simulink model "Computed_Torque_Control"  (R2018b)
settings: Solver=FixedStepAuto  StartTime=0.0  StopTime=5  FixedStep=0.0005  RelTol=1e-3
model workspace (MAT data in the model file):
  Ball.radius = 0.03
  Ball.density = 1000
  Plane.length = 1
  Plane.width = 1
  Plane.depth = 0.1
  SCARA_Robot = robotics.RigidBodyTree
  SCARA_Robot.TreeInternal = robotics.manip.internal.RigidBodyTree
  SCARA_Robot.TreeInternal.NumBodies = 7
  SCARA_Robot.TreeInternal.Base = robotics.manip.internal.RigidBody
  SCARA_Robot.TreeInternal.Base.Index = 0
  SCARA_Robot.TreeInternal.Base.NameInternal = 'Base'
  SCARA_Robot.TreeInternal.Base.JointInternal = robotics.Joint
  SCARA_Robot.TreeInternal.Base.JointInternal.Type = 'fixed'
  SCARA_Robot.TreeInternal.Base.JointInternal.VelocityNumber = 0
  SCARA_Robot.TreeInternal.Base.JointInternal.PositionNumber = 0
  SCARA_Robot.TreeInternal.Base.JointInternal.MotionSubspace = [0; 0; 0; 0; 0; 0]
  SCARA_Robot.TreeInternal.Base.JointInternal.NameInternal = 'base_jnt'
  SCARA_Robot.TreeInternal.Base.ParentIndex = -1
  SCARA_Robot.TreeInternal.Base.ChildrenIndices = [1 0 0 0 0 0 1]
  SCARA_Robot.TreeInternal.Base.MassInternal = 1
  SCARA_Robot.TreeInternal.Base.CenterOfMassInternal = [0 0 0]
  SCARA_Robot.TreeInternal.Base.InertiaInternal = [1  0  0; 0  1  0; 0  0  1]
  SCARA_Robot.TreeInternal.Base.SpatialInertia = [1  0  0  0  0  0; 0  1  0  0  0  0; 0  0  1  0  0  0; 0  0  0  1  0  0; 0  0  0  0  1  0; 0  0  0  0  0  1]
  SCARA_Robot.TreeInternal.Gravity = [0 0 -9.80665]
  SCARA_Robot.TreeInternal.Bodies{1} = robotics.manip.internal.RigidBody
  SCARA_Robot.TreeInternal.Bodies{1}.Index = 1
  SCARA_Robot.TreeInternal.Bodies{1}.NameInternal = 'Body1'
  SCARA_Robot.TreeInternal.Bodies{1}.JointInternal = robotics.Joint
  SCARA_Robot.TreeInternal.Bodies{1}.JointInternal.Type = 'revolute'
  SCARA_Robot.TreeInternal.Bodies{1}.JointInternal.VelocityNumber = 1
  SCARA_Robot.TreeInternal.Bodies{1}.JointInternal.PositionNumber = 1
  SCARA_Robot.TreeInternal.Bodies{1}.JointInternal.MotionSubspace = [0; 0; 1; 0; 0; 0]
  SCARA_Robot.TreeInternal.Bodies{1}.JointInternal.InTree = 1
  SCARA_Robot.TreeInternal.Bodies{1}.JointInternal.JointToParentTransform = [1  0  0  0; 0  1  0  0; 0  0  1  0.2335; 0  0  0  1]
  SCARA_Robot.TreeInternal.Bodies{1}.JointInternal.NameInternal = 'Joint1'
  SCARA_Robot.TreeInternal.Bodies{1}.JointInternal.PositionLimitsInternal = [-3.14159265359 3.14159265359]
  SCARA_Robot.TreeInternal.Bodies{1}.JointInternal.JointAxisInternal = [0 0 1]
  SCARA_Robot.TreeInternal.Bodies{1}.ParentIndex = 0
  SCARA_Robot.TreeInternal.Bodies{1}.ChildrenIndices = [0 1]
  SCARA_Robot.TreeInternal.Bodies{1}.MassInternal = 3.12934702863
  SCARA_Robot.TreeInternal.Bodies{1}.CenterOfMassInternal = [0.108937389495 0 0.0763962080079]
  SCARA_Robot.TreeInternal.Bodies{1}.InertiaInternal = [0.0248122549552  -1.93363586828e-20  -0.0276846659585; -1.93363586828e-20  0.092692509819  4.00877355014e-19; -0.0276846659585  4.00877355014e-19  0.0776265146367]
  SCARA_Robot.TreeInternal.Bodies{1}.SpatialInertia = [0.0248122549552  -1.93363586828e-20  -0.0276846659585  0  -0.239070246528  0; -1.93363586828e-20  0.092692509819  4.00877355014e-19  0.239070246528  0  -0.340902896122; -0.0276846659585  4.00877355014e-19  0.0776265146367  0  0.340902896122  0; 0  0.239070246528  0  3.12934702863  0  0; -0.239070246528  0  0.340902896122  0  3.12934702863  0; 0  -0.340902896122  0  0  0  3.12934702863]
  SCARA_Robot.TreeInternal.Bodies{2} = robotics.manip.internal.RigidBody
  SCARA_Robot.TreeInternal.Bodies{2}.Index = 2
  SCARA_Robot.TreeInternal.Bodies{2}.NameInternal = 'Body2'
  SCARA_Robot.TreeInternal.Bodies{2}.JointInternal = robotics.Joint
  SCARA_Robot.TreeInternal.Bodies{2}.JointInternal.Type = 'revolute'
  SCARA_Robot.TreeInternal.Bodies{2}.JointInternal.VelocityNumber = 1
  SCARA_Robot.TreeInternal.Bodies{2}.JointInternal.PositionNumber = 1
  SCARA_Robot.TreeInternal.Bodies{2}.JointInternal.MotionSubspace = [0; 0; 1; 0; 0; 0]
  SCARA_Robot.TreeInternal.Bodies{2}.JointInternal.InTree = 1
  SCARA_Robot.TreeInternal.Bodies{2}.JointInternal.JointToParentTransform = [1  0  0  0.25; 0  1  0  0; 0  0  1  0.09; 0  0  0  1]
  SCARA_Robot.TreeInternal.Bodies{2}.JointInternal.NameInternal = 'Joint2'
  SCARA_Robot.TreeInternal.Bodies{2}.JointInternal.PositionLimitsInternal = [-3.14159265359 3.14159265359]
  SCARA_Robot.TreeInternal.Bodies{2}.JointInternal.JointAxisInternal = [0 0 1]
  SCARA_Robot.TreeInternal.Bodies{2}.ParentIndex = 1
  SCARA_Robot.TreeInternal.Bodies{2}.ChildrenIndices = [0 0 1]
  SCARA_Robot.TreeInternal.Bodies{2}.MassInternal = 2.8
  SCARA_Robot.TreeInternal.Bodies{2}.CenterOfMassInternal = [0.0730251626831 0 0.08]
  SCARA_Robot.TreeInternal.Bodies{2}.InertiaInternal = [0.0343024465413  9.77217250727e-20  -0.016902140627; 9.77217250727e-20  0.0618863054598  -9.17919345749e-19; -0.016902140627  -9.17919345749e-19  0.0363706015866]
  SCARA_Robot.TreeInternal.Bodies{2}.SpatialInertia = [0.0343024465413  9.77217250727e-20  -0.016902140627  0  -0.224  0; 9.77217250727e-20  0.0618863054598  -9.17919345749e-19  0.224  0  -0.204470455513; -0.016902140627  -9.17919345749e-19  0.0363706015866  0  0.204470455513  0; 0  0.224  0  2.8  0  0; -0.224  0  0.204470455513  0  2.8  0; 0  -0.204470455513  0  0  0  2.8]
  SCARA_Robot.TreeInternal.Bodies{3} = robotics.manip.internal.RigidBody
  SCARA_Robot.TreeInternal.Bodies{3}.Index = 3
  SCARA_Robot.TreeInternal.Bodies{3}.NameInternal = 'Body3'
  SCARA_Robot.TreeInternal.Bodies{3}.JointInternal = robotics.Joint
  SCARA_Robot.TreeInternal.Bodies{3}.JointInternal.Type = 'prismatic'
  SCARA_Robot.TreeInternal.Bodies{3}.JointInternal.VelocityNumber = 1
  SCARA_Robot.TreeInternal.Bodies{3}.JointInternal.PositionNumber = 1
  SCARA_Robot.TreeInternal.Bodies{3}.JointInternal.MotionSubspace = [0; 0; 0; 0; 0; 1]
  SCARA_Robot.TreeInternal.Bodies{3}.JointInternal.InTree = 1
  SCARA_Robot.TreeInternal.Bodies{3}.JointInternal.JointToParentTransform = [1  0  0  0.142; 0  1  0  -0.008; 0  0  1  0.25; 0  0  0  1]
  SCARA_Robot.TreeInternal.Bodies{3}.JointInternal.NameInternal = 'Joint3'
  SCARA_Robot.TreeInternal.Bodies{3}.JointInternal.PositionLimitsInternal = [-0.5 0.5]
  SCARA_Robot.TreeInternal.Bodies{3}.JointInternal.JointAxisInternal = [0 0 1]
  SCARA_Robot.TreeInternal.Bodies{3}.ParentIndex = 2
  SCARA_Robot.TreeInternal.Bodies{3}.ChildrenIndices = [0 0 0 1]
  SCARA_Robot.TreeInternal.Bodies{3}.MassInternal = 0.0658123859659
  SCARA_Robot.TreeInternal.Bodies{3}.CenterOfMassInternal = [0.008 0.008 -0.161652320553]
  SCARA_Robot.TreeInternal.Bodies{3}.InertiaInternal = [0.00223249562485  -4.21199270182e-06  8.51097993001e-05; -4.21199270182e-06  0.00223249562485  8.51097993001e-05; 8.51097993001e-05  8.51097993001e-05  1.08030484212e-05]
  SCARA_Robot.TreeInternal.Bodies{3}.SpatialInertia = [0.00223249562485  -4.21199270182e-06  8.51097993001e-05  0  0.0106387249125  0.000526499087728; -4.21199270182e-06  0.00223249562485  8.51097993001e-05  -0.0106387249125  0  -0.000526499087728; 8.51097993001e-05  8.51097993001e-05  1.08030484212e-05  -0.000526499087728  0.000526499087728  0; 0  -0.0106387249125  -0.000526499087728  0.0658123859659  0  0; 0.0106387249125  0  0.000526499087728  0  0.0658123859659  0; 0.000526499087728  -0.000526499087728  0  0  0  0.0658123859659]
  SCARA_Robot.TreeInternal.Bodies{4} = robotics.manip.internal.RigidBody
  SCARA_Robot.TreeInternal.Bodies{4}.Index = 4
  SCARA_Robot.TreeInternal.Bodies{4}.NameInternal = 'Body4'
  SCARA_Robot.TreeInternal.Bodies{4}.JointInternal = robotics.Joint
  SCARA_Robot.TreeInternal.Bodies{4}.JointInternal.Type = 'revolute'
  SCARA_Robot.TreeInternal.Bodies{4}.JointInternal.VelocityNumber = 1
  SCARA_Robot.TreeInternal.Bodies{4}.JointInternal.PositionNumber = 1
  SCARA_Robot.TreeInternal.Bodies{4}.JointInternal.MotionSubspace = [0; 0; 1; 0; 0; 0]
  SCARA_Robot.TreeInternal.Bodies{4}.JointInternal.InTree = 1
  SCARA_Robot.TreeInternal.Bodies{4}.JointInternal.JointToParentTransform = [1  0  0  0.008; 0  1  0  0.008; 0  0  1  -0.02; 0  0  0  1]
  SCARA_Robot.TreeInternal.Bodies{4}.JointInternal.NameInternal = 'Joint4'
  SCARA_Robot.TreeInternal.Bodies{4}.JointInternal.PositionLimitsInternal = [-3.14159265359 3.14159265359]
  SCARA_Robot.TreeInternal.Bodies{4}.JointInternal.JointAxisInternal = [0 0 1]
  SCARA_Robot.TreeInternal.Bodies{4}.ParentIndex = 3
  SCARA_Robot.TreeInternal.Bodies{4}.ChildrenIndices = [0 0 0 0 1]
  SCARA_Robot.TreeInternal.Bodies{4}.MassInternal = 0.0638828919245
  SCARA_Robot.TreeInternal.Bodies{4}.CenterOfMassInternal = [-0.000115977158264 0 -0.314685264828]
  SCARA_Robot.TreeInternal.Bodies{4}.InertiaInternal = [0.00634242429346  0  -2.33382122413e-06; 0  0.0063422366579  0; -2.33382122413e-06  0  2.29864595889e-05]
  SCARA_Robot.TreeInternal.Bodies{4}.SpatialInertia = [0.00634242429346  0  -2.33382122413e-06  0  0.0201030047632  0; 0  0.0063422366579  0  -0.0201030047632  0  7.40895626708e-06; -2.33382122413e-06  0  2.29864595889e-05  0  -7.40895626708e-06  0; 0  -0.0201030047632  0  0.0638828919245  0  0; 0.0201030047632  0  -7.40895626708e-06  0  0.0638828919245  0; 0  7.40895626708e-06  0  0  0  0.0638828919245]
  SCARA_Robot.TreeInternal.Bodies{5} = robotics.manip.internal.RigidBody
  SCARA_Robot.TreeInternal.Bodies{5}.Index = 5
  SCARA_Robot.TreeInternal.Bodies{5}.NameInternal = 'Body5'
  SCARA_Robot.TreeInternal.Bodies{5}.JointInternal = robotics.Joint
  SCARA_Robot.TreeInternal.Bodies{5}.JointInternal.Type = 'fixed'
  SCARA_Robot.TreeInternal.Bodies{5}.JointInternal.VelocityNumber = 0
  SCARA_Robot.TreeInternal.Bodies{5}.JointInternal.PositionNumber = 0
  SCARA_Robot.TreeInternal.Bodies{5}.JointInternal.MotionSubspace = [0; 0; 0; 0; 0; 0]
  SCARA_Robot.TreeInternal.Bodies{5}.JointInternal.InTree = 1
  SCARA_Robot.TreeInternal.Bodies{5}.JointInternal.JointToParentTransform = [1  0  0  -2.71050543121e-20; 0  1  0  0; 0  0  1  -0.33; 0  0  0  1]
  SCARA_Robot.TreeInternal.Bodies{5}.JointInternal.NameInternal = 'Joint5'
  SCARA_Robot.TreeInternal.Bodies{5}.ParentIndex = 4
  SCARA_Robot.TreeInternal.Bodies{5}.ChildrenIndices = [0 0 0 0 0 1]
  SCARA_Robot.TreeInternal.Bodies{5}.MassInternal = 0
  SCARA_Robot.TreeInternal.Bodies{5}.CenterOfMassInternal = [0 0 0]
  SCARA_Robot.TreeInternal.Bodies{5}.InertiaInternal = [0  0  0; 0  0  0; 0  0  0]
  SCARA_Robot.TreeInternal.Bodies{5}.SpatialInertia = [0  0  0  0  0  0; 0  0  0  0  0  0; 0  0  0  0  0  0; 0  0  0  0  0  0; 0  0  0  0  0  0; 0  0  0  0  0  0]
  SCARA_Robot.TreeInternal.Bodies{6} = robotics.manip.internal.RigidBody
  SCARA_Robot.TreeInternal.Bodies{6}.Index = 6
  SCARA_Robot.TreeInternal.Bodies{6}.NameInternal = 'Body6'
  SCARA_Robot.TreeInternal.Bodies{6}.JointInternal = robotics.Joint
  SCARA_Robot.TreeInternal.Bodies{6}.JointInternal.Type = 'fixed'
  SCARA_Robot.TreeInternal.Bodies{6}.JointInternal.VelocityNumber = 0
  SCARA_Robot.TreeInternal.Bodies{6}.JointInternal.PositionNumber = 0
  SCARA_Robot.TreeInternal.Bodies{6}.JointInternal.MotionSubspace = [0; 0; 0; 0; 0; 0]
  SCARA_Robot.TreeInternal.Bodies{6}.JointInternal.InTree = 1
  SCARA_Robot.TreeInternal.Bodies{6}.JointInternal.JointToParentTransform = [1  0  0  0; 0  1  0  0; 0  0  1  0; 0  0  0  1]
  SCARA_Robot.TreeInternal.Bodies{6}.JointInternal.NameInternal = 'Joint6'
  SCARA_Robot.TreeInternal.Bodies{6}.ParentIndex = 5
  SCARA_Robot.TreeInternal.Bodies{6}.ChildrenIndices = [0 0 0 0 0]
  SCARA_Robot.TreeInternal.Bodies{6}.MassInternal = 0.113097335529
  SCARA_Robot.TreeInternal.Bodies{6}.CenterOfMassInternal = [0 0 0]
  SCARA_Robot.TreeInternal.Bodies{6}.InertiaInternal = [4.07150407905e-05  0  0; 0  4.07150407905e-05  0; 0  0  4.07150407905e-05]
  SCARA_Robot.TreeInternal.Bodies{6}.SpatialInertia = [4.07150407905e-05  0  0  0  0  0; 0  4.07150407905e-05  0  0  0  0; 0  0  4.07150407905e-05  0  0  0; 0  0  0  0.113097335529  0  0; 0  0  0  0  0.113097335529  0; 0  0  0  0  0  0.113097335529]
  SCARA_Robot.TreeInternal.Bodies{7} = robotics.manip.internal.RigidBody
  SCARA_Robot.TreeInternal.Bodies{7}.Index = 7
  SCARA_Robot.TreeInternal.Bodies{7}.NameInternal = 'Body7'
  SCARA_Robot.TreeInternal.Bodies{7}.JointInternal = robotics.Joint
  SCARA_Robot.TreeInternal.Bodies{7}.JointInternal.Type = 'fixed'
  SCARA_Robot.TreeInternal.Bodies{7}.JointInternal.VelocityNumber = 0
  SCARA_Robot.TreeInternal.Bodies{7}.JointInternal.PositionNumber = 0
  SCARA_Robot.TreeInternal.Bodies{7}.JointInternal.MotionSubspace = [0; 0; 0; 0; 0; 0]
  SCARA_Robot.TreeInternal.Bodies{7}.JointInternal.InTree = 1
  SCARA_Robot.TreeInternal.Bodies{7}.JointInternal.JointToParentTransform = [1  0  0  0; 0  1  0  0; 0  0  1  0; 0  0  0  1]
  SCARA_Robot.TreeInternal.Bodies{7}.JointInternal.NameInternal = 'Joint7'
  SCARA_Robot.TreeInternal.Bodies{7}.ParentIndex = 0
  SCARA_Robot.TreeInternal.Bodies{7}.ChildrenIndices = [0 0 0 0 0 0]
  SCARA_Robot.TreeInternal.Bodies{7}.MassInternal = 0
  SCARA_Robot.TreeInternal.Bodies{7}.CenterOfMassInternal = [0 0 0]
  SCARA_Robot.TreeInternal.Bodies{7}.InertiaInternal = [0  0  0; 0  0  0; 0  0  0]
  SCARA_Robot.TreeInternal.Bodies{7}.SpatialInertia = [0  0  0  0  0  0; 0  0  0  0  0  0; 0  0  0  0  0  0; 0  0  0  0  0  0; 0  0  0  0  0  0; 0  0  0  0  0  0]
  SCARA_Robot.TreeInternal.NumNonFixedBodies = 4
  SCARA_Robot.TreeInternal.PositionNumber = 4
  SCARA_Robot.TreeInternal.VelocityNumber = 4
  SCARA_Robot.TreeInternal.PositionDoFMap = [1  1; 2  2; 3  3; 4  4; 0  -1; 0  -1; 0  -1]
  SCARA_Robot.TreeInternal.VelocityDoFMap = [1  1; 2  2; 3  3; 4  4; 0  -1; 0  -1; 0  -1]
  SCARA_Robot.TreeInternal.MaxNumBodies = 7
  SCARA_Robot.TreeInternal.MaxNameLength = 200
  SCARA_Robot.TreeInternal.MaxJointPositionNumber = 7
  SCARA_Robot.TreeInternal.VisualizationInfo = robotics.manip.internal.VisualizationInfo
  SCARA_Robot.TreeInternal.VisualizationInfo.ShowTag = 'DO_NOT_EDIT_iWX9d'
  SCARA_Robot.TreeInternal.DataFormatInternal = 'struct'
  coff = [1 40 400]
  smiData.RigidTransform(1).translation = [250 0 20]
  smiData.RigidTransform(1).angle = 3.14159265359
  smiData.RigidTransform(1).axis = [1 0 0]
  smiData.RigidTransform(1).ID = 'B[Link1-1:-:Link2-1]'
  smiData.RigidTransform(2).translation = [0 0 270]
  smiData.RigidTransform(2).angle = 3.14159265359
  smiData.RigidTransform(2).axis = [1 0 0]
  smiData.RigidTransform(2).ID = 'F[Link1-1:-:Link2-1]'
  smiData.RigidTransform(3).translation = [0 0 110]
  smiData.RigidTransform(3).angle = 0
  smiData.RigidTransform(3).axis = [0 0 0]
  smiData.RigidTransform(3).ID = 'B[Base-1:-:Link1-1]'
  smiData.RigidTransform(4).translation = [0 0 110]
  smiData.RigidTransform(4).angle = 3.14159265359
  smiData.RigidTransform(4).axis = [1 0 0]
  smiData.RigidTransform(4).ID = 'F[Base-1:-:Link1-1]'
  smiData.RigidTransform(5).translation = [150 0 20]
  smiData.RigidTransform(5).angle = 3.14159265359
  smiData.RigidTransform(5).axis = [1 0 0]
  smiData.RigidTransform(5).ID = 'B[Link2-1:-:Move-1]'
  smiData.RigidTransform(6).translation = [0 0 320]
  smiData.RigidTransform(6).angle = 0
  smiData.RigidTransform(6).axis = [0 0 1]
  smiData.RigidTransform(6).ID = 'F[Link2-1:-:Move-1]'
  smiData.RigidTransform(7).translation = [0 0 300]
  smiData.RigidTransform(7).angle = 3.14159265359
  smiData.RigidTransform(7).axis = [1 0 0]
  smiData.RigidTransform(7).ID = 'B[Move-1:-:Rot-1]'
  smiData.RigidTransform(8).translation = [0 0 -300]
  smiData.RigidTransform(8).angle = 0
  smiData.RigidTransform(8).axis = [0 0 0]
  smiData.RigidTransform(8).ID = 'F[Move-1:-:Rot-1]'
  smiData.RigidTransform(9).translation = [0 0 123.5]
  smiData.RigidTransform(9).angle = 0
  smiData.RigidTransform(9).axis = [0 0 0]
  smiData.RigidTransform(9).ID = 'RootGround[Base-1]'
  smiData.Solid(1).mass = 2.8
  smiData.Solid(1).CoM = [73.0251626831 0 190]
  smiData.Solid(1).MoI = [16382.4465413 29034.8171821 21439.1133089]
  smiData.Solid(1).PoI = [0 544.504186027 0]
  smiData.Solid(1).color = [0.8 0.3 0.3]
  smiData.Solid(1).opacity = 1
  smiData.Solid(1).ID = 'Link2*:*榛樿'
  smiData.Solid(2).mass = 0.0638828919245
  smiData.Solid(2).CoM = [-0.115977158264 0 15.3147351721]
  smiData.Solid(2).MoI = [16.3049156988 16.1164208702 22.9856003192]
  smiData.Solid(2).PoI = [0 -0.00233185912567 0]
  smiData.Solid(2).color = [0.3 0.8 0.3]
  smiData.Solid(2).opacity = 1
  smiData.Solid(2).ID = 'Rot*:*榛樿'
  smiData.Solid(3).mass = 7.54037730286
  smiData.Solid(3).CoM = [0 -12.2090965753 111.939248054]
  smiData.Solid(3).MoI = [67953.4260367 46975.8188154 47346.1777637]
  smiData.Solid(3).PoI = [2150.03105694 0 0]
  smiData.Solid(3).color = [1 0.5 0.8]
  smiData.Solid(3).opacity = 1
  smiData.Solid(3).ID = 'Base*:*榛樿'
  smiData.Solid(4).mass = 3.12934702863
  smiData.Solid(4).CoM = [108.937389495 0 33.6037919921]
  smiData.Solid(4).MoI = [6548.19467291 37291.3779621 40489.4430621]
  smiData.Solid(4).PoI = [0 1640.97739592 0]
  smiData.Solid(4).color = [0.3 0.3 0.5]
  smiData.Solid(4).opacity = 1
  smiData.Solid(4).ID = 'Link1*:*榛樿'
  smiData.Solid(5).mass = 0.0658123859659
  smiData.Solid(5).CoM = [0 0 158.347679447]
  smiData.Solid(5).MoI = [508.509062318 508.509062318 2.37906301758]
  smiData.Solid(5).PoI = [0 0 0]
  smiData.Solid(5).color = [1 0.3 0.3]
  smiData.Solid(5).opacity = 1
  smiData.Solid(5).ID = 'Move*:*榛樿'
  smiData.PrismaticJoint.Pz.Pos = 0
  smiData.PrismaticJoint.ID = '[Link2-1:-:Move-1]'
  smiData.RevoluteJoint(1).Rz.Pos = 90
  smiData.RevoluteJoint(1).ID = '[Link1-1:-:Link2-1]'
  smiData.RevoluteJoint(2).Rz.Pos = 0
  smiData.RevoluteJoint(2).ID = '[Base-1:-:Link1-1]'
  smiData.RevoluteJoint(3).Rz.Pos = 0
  smiData.RevoluteJoint(3).ID = '[Move-1:-:Rot-1]'
values from neighbouring files (symbols this model uses):
  Ball = struct    [SCARA_Robot_DataFile.m]
  Plane = struct    [SCARA_Robot_DataFile.m]
  smiData = struct    [SCARA_Robot_DataFile.m]
undefined symbols (not defined in the file or in its folder): sigbuilder_block, X, Y, Z
libraries: sm_lib x81, nesl_utility x44, robotmaniplib x9, Contact_Forces_Lib x3, Parts_Lib x2, simulink x1
(part 1 of 2)
settings Model: Creator=wqq  LastModifiedBy=wqq

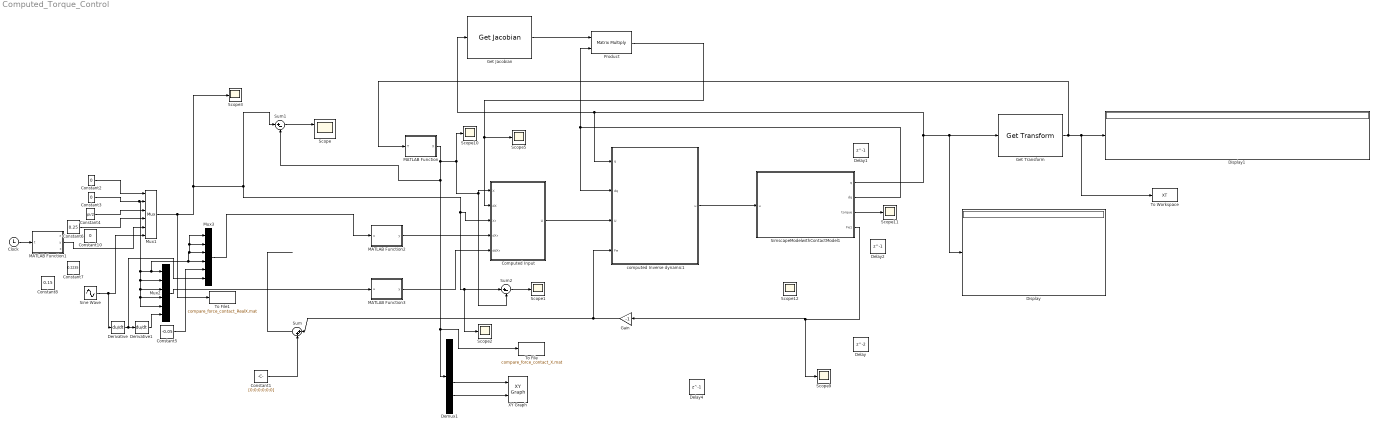
== system Computed_Torque_Control ==
  " Computed Input" : Subsystem
  Clock : Clock
  Constant1 : Constant  Value=[0;0;0;0;0;0]  VectorParams1D=off
  Constant10 : Constant  Value=0
  Constant2 : Constant  Value=0
  Constant3 : Constant  Value=0
  Constant4 : Constant  Value=pi/2
  Constant5 : Constant  Value=-0.05  VectorParams1D=off
  Constant6 : Constant  Value=0.25
  Constant7 : Constant  Value=0.2235
  Constant8 : Constant  Value=0.15
  Delay : Delay
  Delay1 : Delay  DelayLength=1  InitialCondition=[0;pi/2;0;0]
  Delay2 : Delay  DelayLength=1  InitialCondition=[0;0;0;0]
  Delay4 : Delay  DelayLength=1  InitialCondition=[0;0;0;0;0;0]
  Demux1 : Demux  Outputs=6
  Derivative : Derivative
  Derivative1 : Derivative
  Display : Display
  Display1 : Display
  Gain : Gain  Gain=-1
  Get Jacobian : robotmaniplib/Get Jacobian  RigidBodyTree=SCARA_Robot  EndEffector=Body5
      settings: SourceProductName=Robotics System Toolbox
  Get Transform : robotmaniplib/Get Transform  RigidBodyTree=SCARA_Robot  SourceBody=Body5  TargetBody=Body7
      settings: SourceProductName=Robotics System Toolbox
  MATLAB Function : MATLAB Function  TreatAsAtomicUnit=on
  MATLAB Function1 : MATLAB Function  TreatAsAtomicUnit=on
  MATLAB Function2 : MATLAB Function  TreatAsAtomicUnit=on
  MATLAB Function3 : MATLAB Function  TreatAsAtomicUnit=on
  Mux1 : Mux  Inputs=6
  Mux2 : Mux  Inputs=6
  Mux3 : Mux  Inputs=6
  Product : Product  Multiplication=Matrix(*)
  Scope : Scope  NumInputPorts=2
  Scope{1..3,5,9..12} (8 alike) : Scope
  SimscapeModelwithContactModel1 : Subsystem
      mask Display: image('SCARA_picture.png');
  Sine Wave : Sin  Amplitude=0.5  Bias=0.2235  Frequency=3  SampleTime=0
  Sum : Sum  Inputs=|++
  Sum1 : Sum  Inputs=|+-
  Sum2 : Sum  Inputs=|+-
  To File : ToFile  Filename=compare_force_contact_X.mat  MatrixName=X  SaveFormat=Timeseries
  To File1 : ToFile  Filename=compare_force_contact_RealX.mat  MatrixName=RealX  SaveFormat=Timeseries
  To Workspace : ToWorkspace  VariableName=XT  SaveFormat=Timeseries  SampleTime=-1
  XY Graph : simulink/Sinks/XY Graph  xmin=0.1  xmax=0.4  ymin=-0.4  ymax=0.4  st=-1
  computed Inverse dynamic1 : Subsystem
  wires:
  Derivative1/1 -> Mux2/6
  MATLAB Function1/2(y) -> Mux1/5
  Derivative/1 -> Mux3/6, Derivative1/1
  SimscapeModelwithContactModel1/2(dq) -> computed Inverse dynamic1/2(dq), Product/2
  Constant1/1 -> Sum/2
  Constant6/1 -> Mux1/4
  Gain/1 -> computed Inverse dynamic1/4(Fe), Sum/1
  SimscapeModelwithContactModel1/4(Fe1) -> Gain/1, Scope9/1
  SimscapeModelwithContactModel1/1(q) -> Display/1, Get Transform/1, computed Inverse dynamic1/1(q), Get Jacobian/1
  Sum/1 -> ?
  Sum1/1 -> Scope/1
  Demux1/4 -> XY Graph/1
  computed Inverse dynamic1/1(u) -> SimscapeModelwithContactModel1/1(u)
  MATLAB Function/1(X) -> Sum1/2, To File/1, Demux1/1, Scope10/1, " Computed Input"/1(X), Sum2/2
  Mux2/1 -> MATLAB Function3/1(u)
  Sum2/1 -> Scope1/1
  Demux1/5 -> XY Graph/2
  Mux1/1 -> To File1/1, Scope3/1, Scope2/1, Sum2/1, " Computed Input"/3(Xr), Sum1/1
  Constant2/1 -> Mux1/1
  " Computed Input"/1(U) -> computed Inverse dynamic1/3(U)
  Constant3/1 -> Mux1/2, Mux3/1, Mux3/2, Mux3/3, Mux3/4, Mux2/1, Mux2/2, Mux2/3, Mux2/4, Mux2/5
  Get Transform/1 -> MATLAB Function/1(T), To Workspace/1, Display1/1
  SimscapeModelwithContactModel1/3(torque) -> Scope11/1
  Sine Wave/1 -> Derivative/1, Mux1/6
  Product/1 -> Scope5/1, " Computed Input"/2(dX)
  Constant4/1 -> Mux1/3
  Constant5/1 -> Mux3/5
  Get Jacobian/1 -> Product/1
  Clock/1 -> MATLAB Function1/1(t)
  Mux3/1 -> MATLAB Function2/1(u)
  MATLAB Function2/1(y) -> " Computed Input"/4(dXr)
  MATLAB Function3/1(y) -> " Computed Input"/5(ddXr)

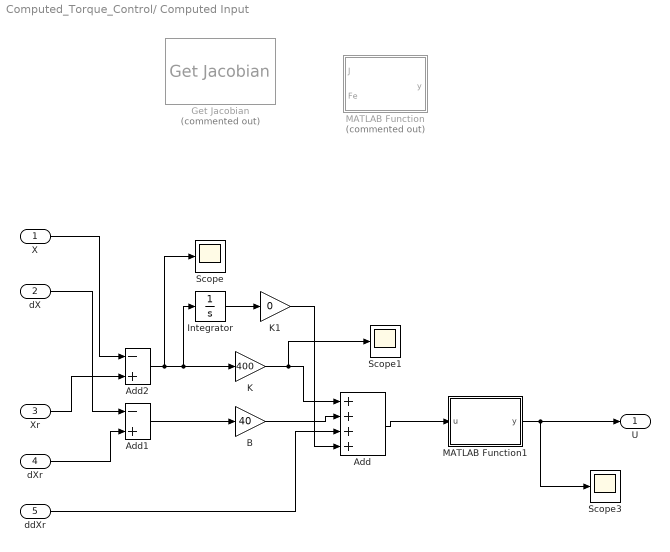
== system Computed_Torque_Control/ Computed Input ==
  X : Inport
  dX : Inport  Port=2
  Xr : Inport  Port=3
  dXr : Inport  Port=4
  ddXr : Inport  Port=5
  Add : Sum  Inputs=++++
  Add1 : Sum  Inputs=-+
  Add2 : Sum  Inputs=-+
  B : Gain  Gain=40
  Get Jacobian : robotmaniplib/Get Jacobian  Commented=on  RigidBodyTree=SCARA_Robot  EndEffector=Body5
      settings: SourceProductName=Robotics System Toolbox
  Integrator : Integrator
  K : Gain  Gain=400
  K1 : Gain  Gain=0
  MATLAB Function : MATLAB Function  Commented=on  TreatAsAtomicUnit=on
  MATLAB Function1 : MATLAB Function  TreatAsAtomicUnit=on
  Scope : Scope
  Scope1 : Scope
  Scope3 : Scope
  U : Outport
  wires:
  ddXr/1 -> Add/3
  dXr/1 -> Add1/2
  dX/1 -> Add1/1
  B/1 -> Add/2
  Xr/1 -> Add2/2
  K/1 -> Scope1/1, Add/1
  Add/1 -> MATLAB Function1/1(u)
  X/1 -> Add2/1
  Add2/1 -> Integrator/1, K/1, Scope/1
  Add1/1 -> B/1
  MATLAB Function1/1(y) -> U/1, Scope3/1
  Integrator/1 -> K1/1
  K1/1 -> Add/4

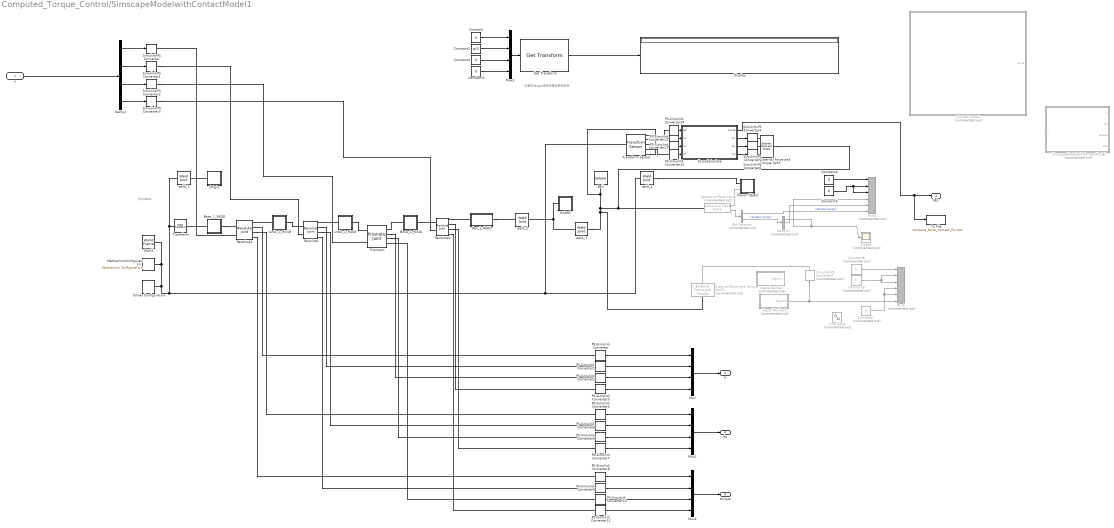
== system Computed_Torque_Control/SimscapeModelwithContactModel1 ==
  note: 这里的target坐标系是世界坐标系
  note: Myrobot
  u : Inport
  Ball : Parts_Lib/Sphere  Tag=CustomStyle  sph_radius=Ball.radius  sph_density=Ball.density  sph_color=red  sph_opacity=1  mark_type=Rings on center planes  arc_width=[40 50]  arc_angle=60  ring_width=5  ring_irad=0.95  mark_color=axes  mark_opacity_x=1  mark_opacity_y=1  mark_opacity_z=1  mark_opacity=1  ring_opacity=0  arc_opacity=0  arc_extr_data=0
  Base_1_RIGID : Subsystem
  Bus Selector : BusSelector  Commented=on  OutputSignals=Normal Force,Friction Force
  Constant{,2..5} (5 alike) : Constant  Value=0
  Constant1 : Constant  Value=pi/2
  Constant6 : Constant  Commented=on  Value=0
  Constant7 : Constant  Commented=on  Value=0
  Constant8 : Constant  Commented=on  Value=0
  Contact Force1 : Subsystem  Commented=on
  Demux : Demux
  Demux1 : Demux  Commented=on  Outputs=3
  Display : Display
  EndEff : Subsystem
  External Force and Torque SphF : sm_lib/Forces and Torques/External Force and Torque  ForceResolutionFrame=AttachedFrame  EnableForceX=on  EnableForceY=on  EnableForceZ=on  EnableForce=off  TorqueResolutionFrame=AttachedFrame  EnableTorqueX=off  EnableTorqueY=off  EnableTorqueZ=off  EnableTorque=off
  External Force and Torque SphF1 : sm_lib/Forces and Torques/External Force and Torque  Commented=on  ForceResolutionFrame=World  EnableForceX=off  EnableForceY=off  EnableForceZ=on  EnableForce=off  TorqueResolutionFrame=AttachedFrame  EnableTorqueX=off  EnableTorqueY=off  EnableTorqueZ=off  EnableTorque=off
  ForceCalculate : Subsystem
  Get Transform : robotmaniplib/Get Transform  RigidBodyTree=SCARA_Robot  SourceBody=Body5  TargetBody=Body7
      settings: SourceProductName=Robotics System Toolbox
  Link1_1_RIGID : Subsystem
  Link2_1_RIGID : Subsystem
  MechanismConfiguration : sm_lib/Utilities/Mechanism Configuration  UniformGravity=Constant  GravityVector=[0 0 -9.80665]  GravityUnits=m/s^2  LinearizationDelta=0.001
  Move_1_RIGID : Subsystem
  Mux{,1..3} (4 alike) : Mux
  Mux4 : Mux  Commented=on  Inputs=6
  Mux5 : Mux  Commented=on  Inputs=6
  Origin : Subsystem
  PS-Simulink Converter{,1..11} (12 alike) : nesl_utility/PS-Simulink Converter  PhysicalDomain=network_engine_domain  SubClassName=ps_output  LeftPortType=input  RightPortType=output  PseudoPeriodic=off  Frequencies=[]  Unit=1  AffineConversion=off
  PS-Simulink Converter12 : nesl_utility/PS-Simulink Converter  PhysicalDomain=network_engine_domain  SubClassName=ps_output  LeftPortType=input  RightPortType=output  PseudoPeriodic=off  Frequencies=[]  Unit=m/s  AffineConversion=off
  PS-Simulink Converter13 : nesl_utility/PS-Simulink Converter  PhysicalDomain=network_engine_domain  SubClassName=ps_output  LeftPortType=input  RightPortType=output  PseudoPeriodic=off  Frequencies=[]  Unit=m/s  AffineConversion=off
  PS-Simulink Converter14 : nesl_utility/PS-Simulink Converter  PhysicalDomain=network_engine_domain  SubClassName=ps_output  LeftPortType=input  RightPortType=output  PseudoPeriodic=off  Frequencies=[]  Unit=m/s  AffineConversion=off
  PS-Simulink Converter29 : nesl_utility/PS-Simulink Converter  PhysicalDomain=network_engine_domain  SubClassName=ps_output  LeftPortType=input  RightPortType=output  PseudoPeriodic=off  Frequencies=[]  Unit=m  AffineConversion=off
  Planar Object : Subsystem
  Prismatic : sm_lib/Joints/Prismatic Joint  SenseConstraintForce=off  SenseConstraintForceX=off  SenseConstraintForceY=off  SenseConstraintForceZ=off  SenseConstraintTorque=off  SenseConstraintTorqueX=off  SenseConstraintTorqueY=off  SenseConstraintTorqueZ=off  SenseTotalForce=off  SenseTotalForceX=off  SenseTotalForceY=off  SenseTotalForceZ=off  SenseTotalTorque=off  SenseTotalTorqueX=off  SenseTotalTorqueY=off  SenseTotalTorqueZ=off  CompositeWrenchDir=FollowerOnBase  CompositeWrenchFrame=BaseFrame  EquilibriumPosition=0  EquilibriumPositionUnits=m  SpringStiffness=0  SpringStiffnessUnits=N/m  DampingCoefficient=0  DampingCoefficientUnits=N/(m/s)  TorqueActuationMode=InputTorque  MotionActuationMode=ComputedMotion  SensePosition=on  SenseVelocity=on  SenseAcceleration=off  SenseTorqueForce=on  PositionTargetSpecify=on  PositionTargetPriority=High  PositionTargetValue=smiData.PrismaticJoint(1).Pz.Pos  PositionTargetValueUnits=m  VelocityTargetSpecify=off  VelocityTargetPriority=High  VelocityTargetValue=0  VelocityTargetValueUnits=m/s
  Revolute : sm_lib/Joints/Revolute Joint  SenseConstraintForce=off  SenseConstraintForceX=off  SenseConstraintForceY=off  SenseConstraintForceZ=off  SenseConstraintTorque=off  SenseConstraintTorqueX=off  SenseConstraintTorqueY=off  SenseConstraintTorqueZ=off  SenseTotalForce=off  SenseTotalForceX=off  SenseTotalForceY=off  SenseTotalForceZ=off  SenseTotalTorque=off  SenseTotalTorqueX=off  SenseTotalTorqueY=off  SenseTotalTorqueZ=off  CompositeWrenchDir=FollowerOnBase  CompositeWrenchFrame=BaseFrame  EquilibriumPosition=0  EquilibriumPositionUnits=rad  SpringStiffness=0  SpringStiffnessUnits=N*m/rad  DampingCoefficient=0  DampingCoefficientUnits=N*m/(rad/s)  TorqueActuationMode=InputTorque  MotionActuationMode=ComputedMotion  SensePosition=on  SenseVelocity=on  SenseAcceleration=off  SenseTorqueForce=on  PositionTargetSpecify=on  PositionTargetPriority=High  PositionTargetValue=smiData.RevoluteJoint(1).Rz.Pos  PositionTargetValueUnits=deg  VelocityTargetSpecify=off  VelocityTargetPriority=High  VelocityTargetValue=0  VelocityTargetValueUnits=deg/s
  Revolute1 : sm_lib/Joints/Revolute Joint  SenseConstraintForce=off  SenseConstraintForceX=off  SenseConstraintForceY=off  SenseConstraintForceZ=off  SenseConstraintTorque=off  SenseConstraintTorqueX=off  SenseConstraintTorqueY=off  SenseConstraintTorqueZ=off  SenseTotalForce=off  SenseTotalForceX=off  SenseTotalForceY=off  SenseTotalForceZ=off  SenseTotalTorque=off  SenseTotalTorqueX=off  SenseTotalTorqueY=off  SenseTotalTorqueZ=off  CompositeWrenchDir=FollowerOnBase  CompositeWrenchFrame=BaseFrame  EquilibriumPosition=0  EquilibriumPositionUnits=rad  SpringStiffness=0  SpringStiffnessUnits=N*m/rad  DampingCoefficient=0  DampingCoefficientUnits=N*m/(rad/s)  TorqueActuationMode=InputTorque  MotionActuationMode=ComputedMotion  SensePosition=on  SenseVelocity=on  SenseAcceleration=off  SenseTorqueForce=on  PositionTargetSpecify=on  PositionTargetPriority=High  PositionTargetValue=smiData.RevoluteJoint(2).Rz.Pos  PositionTargetValueUnits=deg  VelocityTargetSpecify=off  VelocityTargetPriority=High  VelocityTargetValue=0  VelocityTargetValueUnits=deg/s
  Revolute2 : sm_lib/Joints/Revolute Joint  SenseConstraintForce=off  SenseConstraintForceX=off  SenseConstraintForceY=off  SenseConstraintForceZ=off  SenseConstraintTorque=off  SenseConstraintTorqueX=off  SenseConstraintTorqueY=off  SenseConstraintTorqueZ=off  SenseTotalForce=off  SenseTotalForceX=off  SenseTotalForceY=off  SenseTotalForceZ=off  SenseTotalTorque=off  SenseTotalTorqueX=off  SenseTotalTorqueY=off  SenseTotalTorqueZ=off  CompositeWrenchDir=FollowerOnBase  CompositeWrenchFrame=BaseFrame  EquilibriumPosition=0  EquilibriumPositionUnits=rad  SpringStiffness=0  SpringStiffnessUnits=N*m/rad  DampingCoefficient=0  DampingCoefficientUnits=N*m/(rad/s)  TorqueActuationMode=InputTorque  MotionActuationMode=ComputedMotion  SensePosition=on  SenseVelocity=on  SenseAcceleration=off  SenseTorqueForce=on  PositionTargetSpecify=on  PositionTargetPriority=High  PositionTargetValue=smiData.RevoluteJoint(3).Rz.Pos  PositionTargetValueUnits=deg  VelocityTargetSpecify=off  VelocityTargetPriority=High  VelocityTargetValue=0  VelocityTargetValueUnits=deg/s
  Rot_1_RIGID : Subsystem
  Scope1 : Scope  Commented=on
  Signal Builder : Subsystem  Tag=STV Subsys  Commented=on  LoadFcn=sigbuilder_block('load');  StartFcn=sigbuilder_block('start');  StopFcn=sigbuilder_block('stop');  ClipboardFcn=sigbuilder_block('clipboard');  mask(Sigbuilder block){tuvar=[0:10]}
      mask help: Simulink:masks:SigbuilderBlock_MD
      mask init:
      | if ~strcmp(get_param(bdroot(gcbh),'SimulationStatus'),'stopped') tuvar = sigbuilder_block('maskInit'); end
      settings: CopyFcn=sigbuilder_block('copy');  DeleteFcn=sigbuilder_block('delete');  ModelCloseFcn=sigbuilder_block('modelClose');  PreSaveFcn=sigbuilder_block('preSave');  PauseFcn=sigbuilder_block('pause');  ContinueFcn=sigbuilder_block('continue');  NameChangeFcn=sigbuilder_block('namechange');  OpenFcn=sigbuilder_block('open',[437.6 199.2 550.4 400 ]);  CloseFcn=sigbuilder_block('close');
      mask Display: plot(0, 0, 100, 100,[2, 2, 32, 32, 2], [68, 8, 8, 68, 68],[32, 2], [38, 38], [32, 19, 2],[53, 60, 44], [32, 17, 17, 2],[16, 16, 31, 31]);txt = getActiveGroup(gcbh);text(2, 100, txt,'verticalAlignment', 'top');
  Signal Builder1 : Subsystem  Tag=STV Subsys  Commented=on  LoadFcn=sigbuilder_block('load');  StartFcn=sigbuilder_block('start');  StopFcn=sigbuilder_block('stop');  ClipboardFcn=sigbuilder_block('clipboard');  mask(Sigbuilder block){tuvar=[0:10]}
      mask help: Simulink:masks:SigbuilderBlock_MD
      mask init:
      | if ~strcmp(get_param(bdroot(gcbh),'SimulationStatus'),'stopped') tuvar = sigbuilder_block('maskInit'); end
      settings: CopyFcn=sigbuilder_block('copy');  DeleteFcn=sigbuilder_block('delete');  ModelCloseFcn=sigbuilder_block('modelClose');  PreSaveFcn=sigbuilder_block('preSave');  PauseFcn=sigbuilder_block('pause');  ContinueFcn=sigbuilder_block('continue');  NameChangeFcn=sigbuilder_block('namechange');  OpenFcn=sigbuilder_block('open',[437.6 199.2 550.4 400 ]);  CloseFcn=sigbuilder_block('close');
      mask Display: plot(0, 0, 100, 100,[2, 2, 32, 32, 2], [68, 8, 8, 68, 68],[32, 2], [38, 38], [32, 19, 2],[53, 60, 44], [32, 17, 17, 2],[16, 16, 31, 31]);txt = getActiveGroup(gcbh);text(2, 100, txt,'verticalAlignment', 'top');
  SimscapeModelwithContactModel : Subsystem  Commented=on
  Simulink-PS Converter{,1..6} (7 alike) : nesl_utility/Simulink-PS Converter  PhysicalDomain=network_engine_domain  SubClassName=ps_input  LeftPortType=input  RightPortType=output  PseudoPeriodic=off  Frequencies=[]  NoiseDistribution=none  NoiseParameters=[]  Unit=1  AffineConversion=off  FilteringAndDerivatives=provide  SimscapeFilterOrder=1  InputFilterTimeConstant=0.001  UdotUserProvided=0
  Simulink-PS Converter7 : nesl_utility/Simulink-PS Converter  Commented=on  PhysicalDomain=network_engine_domain  SubClassName=ps_input  LeftPortType=input  RightPortType=output  PseudoPeriodic=off  Frequencies=[]  NoiseDistribution=none  NoiseParameters=[]  Unit=1  AffineConversion=off  FilteringAndDerivatives=provide  SimscapeFilterOrder=1  InputFilterTimeConstant=0.001  UdotUserProvided=0
  Sine Wave : Sin  Commented=on  Amplitude=20  SampleTime=0
  Solver Configuration : nesl_utility/Solver Configuration  PhysicalDomain=network_engine_domain  SubClassName=solver  LeftPortType=input  RightPortType=generic  Tones=[]  Harmonics=[]  SimulateNoise=off  Profile=off  UseLocalSampling=off  EnableSwitchedLinearOptims=on  FrequencyDomain=off  UseCCode=off  RelTol=0.001  AbsTol=1e-06  MinStep=1e-09  ToWorkspace=off  RevertToSquareIcSolve=off  NumHomotopyIterations=100  PhasorMode=off  PhasorModeNumHarmonics=1  DoDC=off  ResidualTolerance=1e-09  UseLocalSolver=off  LocalSolverChoice=NE_BACKWARD_EULER_ADVANCER  LocalSolverSampleTime=0.001  DoFixedCost=off  MaxNonlinIter=3  MaxModeIter=2  LinearAlgebra=auto  EquationFormulation=NE_TIME_EF  DelaysMemoryBudget=1024  AutomaticFiltering=on  FilteringTimeConstant=0.001  PartitionStorageMethod=AS_NEEDED  PartitionMemoryBudget=1024
  Sphere to Plane Force : Contact_Forces_Lib/3D/Sphere to Plane Force  Commented=on  sphere_rad=0.03  plane_lenx=1  plane_leny=1  plane_depth=0.1/2  force_law=Linear  k_contact=1e5  b_contact=50  pen_full_damp_F=1e-4  pen_exponent=1  custom_param_1=1  custom_param_2=1  friction_law=Stick-Slip Continuous  mu_kinetic=0.5  mu_static=0.7  v_thr=0.001  vis_on=off  vis_opc_en=0  vis_len_plaBz=0.005  vis_clr=[0.9 0.2 0.2]  vis_opc=0.7
  To File : ToFile  Filename=compare_force_contact_Fe.mat  MatrixName=Fe  SaveFormat=Timeseries
  Transform : sm_lib/Frames and Transforms/Rigid Transform  TranslationMethod=Cartesian  TranslationStandardOffset=0  TranslationLengthUnit=mm  TranslationStandardAxis=+Z  TranslationCartesianOffset=smiData.RigidTransform(9).translation  TranslationROffset=0  TranslationROffsetUnits=m  TranslationZOffset=0  TranslationZOffsetUnits=m  TranslationThetaOffset=0  TranslationThetaOffsetUnits=deg  RotationMethod=ArbitraryAxis  RotationAngleUnits=rad  RotationStandardAxis=+Z  RotationAngle=smiData.RigidTransform(9).angle  RotationArbitraryAxis=smiData.RigidTransform(9).axis  FollAlignAxisA=+X  BaseAlignAxisA=+Y  FollAlignAxisB=+Y  BaseAlignAxisB=+Z  RotationSequenceAxes=FollowerAxes  RotationSequence=XYX  RotationSequenceAngles=[0 0 0]  RotationSequenceAnglesUnits=deg  RotationMatrix=[1 0 0; 0 1 0; 0 0 1]
  Transform Sensor : sm_lib/Frames and Transforms/Transform Sensor  MeasurementFrame=World  SenseAngle=off  SenseAxis=off  SenseAngle1=off  SenseAngle2=off  SenseAngle3=off  SenseQ=off  SenseR=off  SenseOmegaX=off  SenseOmegaY=off  SenseOmegaZ=off  SenseOmega1=off  SenseOmega2=off  SenseOmega3=off  SenseQDot=off  SenseRDot=off  SenseAlphaX=off  SenseAlphaY=off  SenseAlphaZ=off  SenseAlpha1=off  SenseAlpha2=off  SenseAlpha3=off  SenseQDDot=off  SenseRDDot=off  SenseX=off  SenseY=off  SenseZ=on  SenseRad=off  SenseAzim=off  SenseDist=off  SenseInc=off  SenseXDot=on  SenseYDot=on  SenseZDot=on  SenseRadDot=off  SenseAzimDot=off  SenseDistDot=off  SenseIncDot=off  SenseXDDot=off  SenseYDDot=off  SenseZDDot=off  SenseRadDDot=off  SenseAzimDDot=off  SenseDistDDot=off  SenseIncDDot=off
  World : sm_lib/Frames and Transforms/World Frame
  weld_{1..4} (4 alike) : sm_lib/Joints/Weld Joint  SenseConstraintForce=off  SenseConstraintForceX=off  SenseConstraintForceY=off  SenseConstraintForceZ=off  SenseConstraintTorque=off  SenseConstraintTorqueX=off  SenseConstraintTorqueY=off  SenseConstraintTorqueZ=off  SenseTotalForce=off  SenseTotalForceX=off  SenseTotalForceY=off  SenseTotalForceZ=off  SenseTotalTorque=off  SenseTotalTorqueX=off  SenseTotalTorqueY=off  SenseTotalTorqueZ=off  CompositeWrenchDir=FollowerOnBase  CompositeWrenchFrame=BaseFrame
  q : Outport
  dq : Outport  Port=2
  torque : Outport  Port=3
  Fe1 : Outport  Port=4
  wires:
  Demux/4 -> Simulink-PS Converter3/1
  Mux1/1 -> dq/1
  PS-Simulink Converter10/1 -> Mux2/3
  PS-Simulink Converter8/1 -> Mux2/1
  Demux/1 -> Simulink-PS Converter/1
  PS-Simulink Converter11/1 -> Mux2/4
  PS-Simulink Converter5/1 -> Mux1/2
  PS-Simulink Converter/1 -> Mux/1
  Mux2/1 -> torque/1
  PS-Simulink Converter1/1 -> Mux/2
  Demux/2 -> Simulink-PS Converter1/1
  PS-Simulink Converter9/1 -> Mux2/2
  PS-Simulink Converter6/1 -> Mux1/3
  PS-Simulink Converter7/1 -> Mux1/4
  PS-Simulink Converter4/1 -> Mux1/1
  Mux/1 -> q/1
  PS-Simulink Converter2/1 -> Mux/3
  PS-Simulink Converter3/1 -> Mux/4
  Mux3/1 -> Get Transform/1
  Constant/1 -> Mux3/1
  Constant1/1 -> Mux3/2
  Constant2/1 -> Mux3/3
  Constant3/1 -> Mux3/4
  u/1 -> Demux/1
  Get Transform/1 -> Display/1
  Constant4/1 -> Mux4/1
  Constant5/1 -> Mux4/3, Mux4/2
  PS-Simulink Converter29/1 -> ForceCalculate/1(pZ)
  PS-Simulink Converter12/1 -> ForceCalculate/2(vZ)
  PS-Simulink Converter14/1 -> ForceCalculate/4(vY)
  PS-Simulink Converter13/1 -> ForceCalculate/3(vX)
  Demux/3 -> Simulink-PS Converter2/1
  Sphere to Plane Force/1 -> Bus Selector/1
  Bus Selector/1 -> Mux4/6  "<Normal Force>"
  Bus Selector/2 -> Demux1/1  "<Friction Force>"
  Demux1/2 -> Mux4/5
  Demux1/1 -> Mux4/4, Scope1/1
  Constant8/1 -> Mux5/2, Mux5/3
  Constant6/1 -> Mux5/1
  ForceCalculate/2(Fx) -> Simulink-PS Converter4/1
  ForceCalculate/3(Fy) -> Simulink-PS Converter5/1
  ForceCalculate/4(Fz) -> Simulink-PS Converter6/1
  Signal Builder1/1(Signal 1) -> Simulink-PS Converter7/1, Mux5/6
  Constant7/1 -> Mux5/5, Mux5/4
  ForceCalculate/1(Force) -> To File/1, Fe1/1
  connections:
  Revolute2/RConn3 -- PS-Simulink Converter7/LConn1
  Revolute/RConn2 -- PS-Simulink Converter1/LConn1
  Link2_1_RIGID/LConn1 -- Revolute/RConn1
  Move_1_RIGID/LConn1 -- Prismatic/RConn1
  Link1_1_RIGID/LConn1 -- Revolute1/RConn1
  Base_1_RIGID/LConn1 -- Transform/RConn1
  Revolute2/RConn2 -- PS-Simulink Converter3/LConn1
  Revolute1/LConn2 -- Simulink-PS Converter/RConn1
  Revolute1/RConn3 -- PS-Simulink Converter4/LConn1
  Simulink-PS Converter3/RConn1 -- Revolute2/LConn2
  Revolute1/RConn4 -- PS-Simulink Converter8/LConn1
  Move_1_RIGID/RConn1 -- Revolute2/LConn1
  PS-Simulink Converter/LConn1 -- Revolute1/RConn2
  Revolute/RConn4 -- PS-Simulink Converter9/LConn1
  Link2_1_RIGID/RConn1 -- Prismatic/LConn1
  Base_1_RIGID/RConn1 -- Revolute1/LConn1
  Link1_1_RIGID/RConn1 -- Revolute/LConn1
  Revolute2/RConn1 -- Rot_1_RIGID/LConn1
  Prismatic/RConn2 -- PS-Simulink Converter2/LConn1
  Revolute2/RConn4 -- PS-Simulink Converter11/LConn1
  Simulink-PS Converter2/RConn1 -- Prismatic/LConn2
  Simulink-PS Converter1/RConn1 -- Revolute/LConn2
  Revolute/RConn3 -- PS-Simulink Converter5/LConn1
  Prismatic/RConn3 -- PS-Simulink Converter6/LConn1
  Rot_1_RIGID/RConn1 -- weld_2/LConn1
  EndEff/LConn1 -- weld_2/RConn1 -- weld_3/LConn1
  Origin/LConn1 -- weld_1/RConn1
  Ball/LConn1 -- Transform Sensor/RConn1 -- External Force and Torque SphF1/RConn1 -- weld_3/RConn1 -- Sphere to Plane Force/LConn1 -- External Force and Torque SphF/RConn1
  weld_1/LConn1 -- Transform/LConn1 -- World/RConn1 -- MechanismConfiguration/RConn1 -- Solver Configuration/RConn1 -- Transform Sensor/LConn1 -- weld_4/LConn1
  PS-Simulink Converter29/LConn1 -- Transform Sensor/RConn2
  weld_4/RConn1 -- Planar Object/LConn1
  PS-Simulink Converter10/LConn1 -- Prismatic/RConn4
  Transform Sensor/RConn3 -- PS-Simulink Converter13/LConn1
  Transform Sensor/RConn4 -- PS-Simulink Converter14/LConn1
  Transform Sensor/RConn5 -- PS-Simulink Converter12/LConn1
  Sphere to Plane Force/RConn1 -- Planar Object/LConn2
  Simulink-PS Converter4/RConn1 -- External Force and Torque SphF/LConn1
  Simulink-PS Converter5/RConn1 -- External Force and Torque SphF/LConn2
  Simulink-PS Converter6/RConn1 -- External Force and Torque SphF/LConn3
  Simulink-PS Converter7/RConn1 -- External Force and Torque SphF1/LConn1

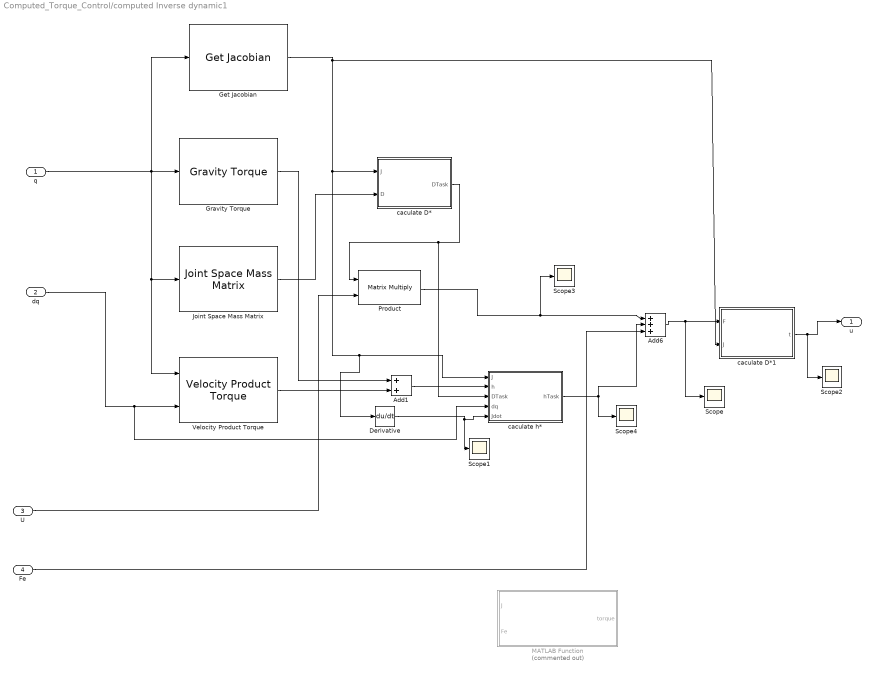
== system Computed_Torque_Control/computed Inverse dynamic1 ==
  q : Inport
  dq : Inport  Port=2
  U : Inport  Port=3
  Fe : Inport  Port=4
  Add1 : Sum
  Add6 : Sum  Inputs=+++
  Derivative : Derivative
  Get Jacobian : robotmaniplib/Get Jacobian  RigidBodyTree=SCARA_Robot  EndEffector=Body5
      settings: SourceProductName=Robotics System Toolbox
  Gravity Torque : robotmaniplib/Gravity Torque  RigidBodyTree=SCARA_Robot
      settings: SourceProductName=Robotics System Toolbox
  Joint Space Mass Matrix : robotmaniplib/Joint Space Mass Matrix  RigidBodyTree=SCARA_Robot
      settings: SourceProductName=Robotics System Toolbox
  MATLAB Function : MATLAB Function  Commented=on  TreatAsAtomicUnit=on
  Product : Product  Multiplication=Matrix(*)
  Scope{,1..4} (5 alike) : Scope
  Velocity Product Torque : robotmaniplib/Velocity Product Torque  RigidBodyTree=SCARA_Robot
      settings: SourceProductName=Robotics System Toolbox
  caculate D* : MATLAB Function  TreatAsAtomicUnit=on
  caculate D*1 : MATLAB Function  TreatAsAtomicUnit=on
  caculate h* : MATLAB Function  TreatAsAtomicUnit=on
  u : Outport
  wires:
  q/1 -> Velocity Product Torque/1, Joint Space Mass Matrix/1, Get Jacobian/1, Gravity Torque/1
  Velocity Product Torque/1 -> Add1/2
  U/1 -> Product/2
  Joint Space Mass Matrix/1 -> caculate D*/2(D)
  Get Jacobian/1 -> Derivative/1, caculate h*/1(J), caculate D*/1(J), caculate D*1/2(J)
  caculate D*/1(DTask) -> caculate h*/3(DTask), Product/1
  Product/1 -> Scope3/1, Add6/1
  Gravity Torque/1 -> Add1/1
  Add1/1 -> caculate h*/2(h)
  dq/1 -> caculate h*/4(dq), Velocity Product Torque/2
  caculate D*1/1(t) -> Scope2/1, u/1
  Add6/1 -> Scope/1, caculate D*1/1(F)
  Derivative/1 -> Scope1/1, caculate h*/5(Jdot)
  caculate h*/1(hTask) -> Add6/2, Scope4/1
  Fe/1 -> Add6/3

== system Computed_Torque_Control/SimscapeModelwithContactModel1/Base_1_RIGID ==
  ReferenceFrame : sm_lib/Frames and Transforms/Reference Frame
  Solid : sm_lib/Body Elements/Solid  InertiaType=Custom  Mass=smiData.Solid(3).mass  MassUnits=kg  CenterOfMass=smiData.Solid(3).CoM  CenterOfMassUnits=mm  MomentsOfInertia=smiData.Solid(3).MoI  MomentsOfInertiaUnits=kg*mm^2  ProductsOfInertia=smiData.Solid(3).PoI  ProductsOfInertiaUnits=kg*mm^2  BasedOnType=Density  Density=1000  DensityUnits=kg/m^3  DoExposeReferenceFrame=off  SerializedFrames=<Frames><Frame><Id>Frame1</Id><Value><Name>F2</Name><Origin><Source>GeometricFeature</Source><FeatureName>cylindrical surface 2</FeatureName></Origin><PrimaryAxis><DefinedDirection>+Z</DefinedDirection><Source>ReferenceFrame</Source><SourceDirection>+Z</SourceDirection><FeatureName></FeatureName></PrimaryAxis><SecondaryAxis><DefinedDirection>+X</DefinedDirection><Source>ReferenceFrame</Source><SourceDirection>+X</SourceDirection><FeatureName></FeatureName></SecondaryAxis></Value></Frame></Frames>  GraphicType=FromGeometry  MarkerShape=Sphere  MarkerSize=10  GraphicVisPropType=SimpleVisualProperties  GraphicDiffuseColor=smiData.Solid(3).color  GraphicSpecularColor=[0.5 0.5 0.5 1.0]  GraphicAmbientColor=[0.15 0.15 0.15 1.0]  GraphicEmissiveColor=[0.0 0.0 0.0 1.0]  GraphicShininess=75  GraphicOpacity=smiData.Solid(3).opacity  GeometryShape=FromFile  RectangleSize=[1 1]  RectangleSizeUnits=m  BrickDimensions=[1 1 1]  BrickDimensionUnits=m  CylinderRadius=1  CylinderRadiusUnits=m  CylinderLength=1  CylinderLengthUnits=m  SphereRadius=1  SphereRadiusUnits=m  EllipsoidRadii=[1 1 1]  EllipsoidRadiiUnits=m  ExtrusionCrossSection=[1 1; -1 1; -1 -1; 1 -1]  ExtrusionCrossSectionUnits=m  ExtrusionLength=1  ExtrusionLengthUnits=m  PolygonNumSides=3  PolygonOuterRadius=1  PolygonOuterRadiusUnits=m  ExtGeomFileType=STEP  ExtGeomFileName=Base_默认_sldprt.STEP  ExtGeomFileUnits=m  RevolutionCrossSection=[1 1; 1 -1; 2 -1; 2 1]  RevolutionCrossSectionUnits=m  RevolutionExtent=Full  RevolutionAngle=180  RevolutionAngleUnits=deg
  Transform : sm_lib/Frames and Transforms/Rigid Transform  TranslationMethod=Cartesian  TranslationStandardOffset=0  TranslationLengthUnit=mm  TranslationStandardAxis=+Z  TranslationCartesianOffset=smiData.RigidTransform(3).translation  TranslationROffset=0  TranslationROffsetUnits=m  TranslationZOffset=0  TranslationZOffsetUnits=m  TranslationThetaOffset=0  TranslationThetaOffsetUnits=deg  RotationMethod=ArbitraryAxis  RotationAngleUnits=rad  RotationStandardAxis=+Z  RotationAngle=smiData.RigidTransform(3).angle  RotationArbitraryAxis=smiData.RigidTransform(3).axis  FollAlignAxisA=+X  BaseAlignAxisA=+Y  FollAlignAxisB=+Y  BaseAlignAxisB=+Z  RotationSequenceAxes=FollowerAxes  RotationSequence=XYX  RotationSequenceAngles=[0 0 0]  RotationSequenceAnglesUnits=deg  RotationMatrix=[1 0 0; 0 1 0; 0 0 1]
  F1 : PMIOPort  Side=Left
  F : PMIOPort  Port=2  Side=Right
  connections:
  ReferenceFrame/RConn1 -- Solid/LConn1 -- Transform/LConn1 -- F1/RConn1
  Transform/RConn1 -- F/RConn1

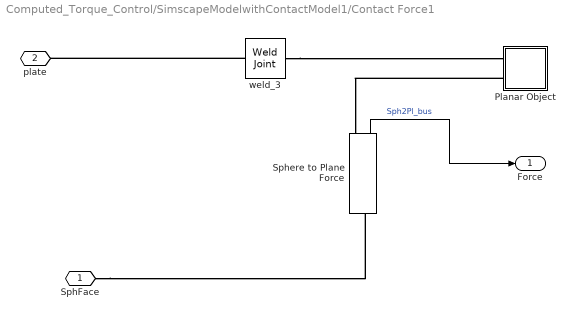
== system Computed_Torque_Control/SimscapeModelwithContactModel1/Contact Force1 ==
  Planar Object : Subsystem
  Sphere to Plane Force : Contact_Forces_Lib/3D/Sphere to Plane Force  sphere_rad=Ball.radius  plane_lenx=Plane.width  plane_leny=Plane.length  plane_depth=0.1/2  force_law=Nonlinear  k_contact=1e7  b_contact=1e3  pen_full_damp_F=1e-4  pen_exponent=1  custom_param_1=1  custom_param_2=1  friction_law=None  mu_kinetic=0.5  mu_static=0.7  v_thr=0.001  vis_on=off  vis_opc_en=0  vis_len_plaBz=Plane.depth*0.1  vis_clr=[0.9 0.2 0.2]  vis_opc=0.7
  weld_3 : sm_lib/Joints/Weld Joint  SenseConstraintForce=off  SenseConstraintForceX=off  SenseConstraintForceY=off  SenseConstraintForceZ=off  SenseConstraintTorque=off  SenseConstraintTorqueX=off  SenseConstraintTorqueY=off  SenseConstraintTorqueZ=off  SenseTotalForce=off  SenseTotalForceX=off  SenseTotalForceY=off  SenseTotalForceZ=off  SenseTotalTorque=off  SenseTotalTorqueX=off  SenseTotalTorqueY=off  SenseTotalTorqueZ=off  CompositeWrenchDir=FollowerOnBase  CompositeWrenchFrame=BaseFrame
  SphFace : PMIOPort  Side=Left
  plate : PMIOPort  Port=2  Side=Left
  Force : Outport
  wires:
  Sphere to Plane Force/1 -> Force/1  "Sph2Pl_bus"
  connections:
  weld_3/RConn1 -- Planar Object/LConn1
  SphFace/RConn1 -- Sphere to Plane Force/LConn1
  weld_3/LConn1 -- plate/RConn1
  Planar Object/LConn2 -- Sphere to Plane Force/RConn1

== system Computed_Torque_Control/SimscapeModelwithContactModel1/EndEff ==
  ReferenceFrame : sm_lib/Frames and Transforms/Reference Frame
  F : PMIOPort  Side=Left
  connections:
  ReferenceFrame/RConn1 -- F/RConn1

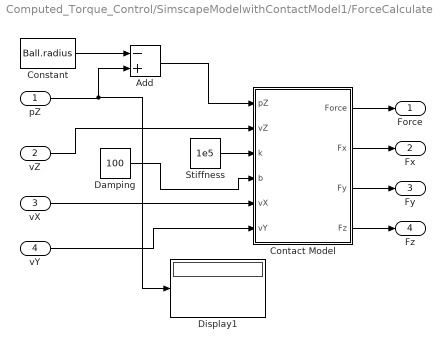
== system Computed_Torque_Control/SimscapeModelwithContactModel1/ForceCalculate ==
  pZ : Inport
  vZ : Inport  Port=2
  vX : Inport  Port=3
  vY : Inport  Port=4
  Add : Sum  Inputs=-+
  Constant : Constant  Value=Ball.radius
  Contact Model : MATLAB Function  TreatAsAtomicUnit=on
  Damping : Constant  Value=100
  Display1 : Display
  Stiffness : Constant  Value=1e5
  Force : Outport
  Fx : Outport  Port=2
  Fy : Outport  Port=3
  Fz : Outport  Port=4
  wires:
  pZ/1 -> Display1/1, Add/2
  vZ/1 -> Contact Model/2(vZ)
  Contact Model/1(Force) -> Force/1
  Stiffness/1 -> Contact Model/3(k)
  Damping/1 -> Contact Model/4(b)
  Constant/1 -> Add/1
  Add/1 -> Contact Model/1(pZ)
  vX/1 -> Contact Model/5(vX)
  vY/1 -> Contact Model/6(vY)
  Contact Model/2(Fx) -> Fx/1
  Contact Model/3(Fy) -> Fy/1
  Contact Model/4(Fz) -> Fz/1

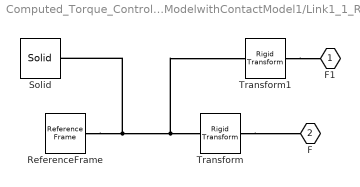
== system Computed_Torque_Control/SimscapeModelwithContactModel1/Link1_1_RIGID ==
  ReferenceFrame : sm_lib/Frames and Transforms/Reference Frame
  Solid : sm_lib/Body Elements/Solid  InertiaType=Custom  Mass=smiData.Solid(4).mass  MassUnits=kg  CenterOfMass=smiData.Solid(4).CoM  CenterOfMassUnits=mm  MomentsOfInertia=smiData.Solid(4).MoI  MomentsOfInertiaUnits=kg*mm^2  ProductsOfInertia=smiData.Solid(4).PoI  ProductsOfInertiaUnits=kg*mm^2  BasedOnType=Density  Density=1000  DensityUnits=kg/m^3  DoExposeReferenceFrame=on  SerializedFrames=<Frames/>  GraphicType=FromGeometry  MarkerShape=Sphere  MarkerSize=10  GraphicVisPropType=SimpleVisualProperties  GraphicDiffuseColor=smiData.Solid(4).color  GraphicSpecularColor=[0.5 0.5 0.5 1.0]  GraphicAmbientColor=[0.15 0.15 0.15 1.0]  GraphicEmissiveColor=[0.0 0.0 0.0 1.0]  GraphicShininess=75  GraphicOpacity=smiData.Solid(4).opacity  GeometryShape=FromFile  RectangleSize=[1 1]  RectangleSizeUnits=m  BrickDimensions=[1 1 1]  BrickDimensionUnits=m  CylinderRadius=1  CylinderRadiusUnits=m  CylinderLength=1  CylinderLengthUnits=m  SphereRadius=1  SphereRadiusUnits=m  EllipsoidRadii=[1 1 1]  EllipsoidRadiiUnits=m  ExtrusionCrossSection=[1 1; -1 1; -1 -1; 1 -1]  ExtrusionCrossSectionUnits=m  ExtrusionLength=1  ExtrusionLengthUnits=m  PolygonNumSides=3  PolygonOuterRadius=1  PolygonOuterRadiusUnits=m  ExtGeomFileType=STEP  ExtGeomFileName=Link1_默认_sldprt.STEP  ExtGeomFileUnits=m  RevolutionCrossSection=[1 1; 1 -1; 2 -1; 2 1]  RevolutionCrossSectionUnits=m  RevolutionExtent=Full  RevolutionAngle=180  RevolutionAngleUnits=deg
  Transform : sm_lib/Frames and Transforms/Rigid Transform  TranslationMethod=Cartesian  TranslationStandardOffset=0  TranslationLengthUnit=mm  TranslationStandardAxis=+Z  TranslationCartesianOffset=smiData.RigidTransform(1).translation  TranslationROffset=0  TranslationROffsetUnits=m  TranslationZOffset=0  TranslationZOffsetUnits=m  TranslationThetaOffset=0  TranslationThetaOffsetUnits=deg  RotationMethod=ArbitraryAxis  RotationAngleUnits=rad  RotationStandardAxis=+Z  RotationAngle=smiData.RigidTransform(1).angle  RotationArbitraryAxis=smiData.RigidTransform(1).axis  FollAlignAxisA=+X  BaseAlignAxisA=+Y  FollAlignAxisB=+Y  BaseAlignAxisB=+Z  RotationSequenceAxes=FollowerAxes  RotationSequence=XYX  RotationSequenceAngles=[0 0 0]  RotationSequenceAnglesUnits=deg  RotationMatrix=[1 0 0; 0 1 0; 0 0 1]
  Transform1 : sm_lib/Frames and Transforms/Rigid Transform  TranslationMethod=Cartesian  TranslationStandardOffset=0  TranslationLengthUnit=mm  TranslationStandardAxis=+Z  TranslationCartesianOffset=smiData.RigidTransform(4).translation  TranslationROffset=0  TranslationROffsetUnits=m  TranslationZOffset=0  TranslationZOffsetUnits=m  TranslationThetaOffset=0  TranslationThetaOffsetUnits=deg  RotationMethod=ArbitraryAxis  RotationAngleUnits=rad  RotationStandardAxis=+Z  RotationAngle=smiData.RigidTransform(4).angle  RotationArbitraryAxis=smiData.RigidTransform(4).axis  FollAlignAxisA=+X  BaseAlignAxisA=+Y  FollAlignAxisB=+Y  BaseAlignAxisB=+Z  RotationSequenceAxes=FollowerAxes  RotationSequence=XYX  RotationSequenceAngles=[0 0 0]  RotationSequenceAnglesUnits=deg  RotationMatrix=[1 0 0; 0 1 0; 0 0 1]
  F1 : PMIOPort  Side=Left
  F : PMIOPort  Port=2  Side=Right
  connections:
  Solid/RConn1 -- Transform/LConn1 -- Transform1/LConn1 -- ReferenceFrame/RConn1
  Transform/RConn1 -- F/RConn1
  Transform1/RConn1 -- F1/RConn1

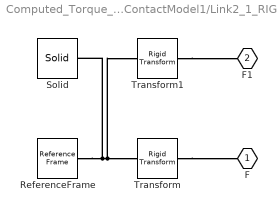
== system Computed_Torque_Control/SimscapeModelwithContactModel1/Link2_1_RIGID ==
  ReferenceFrame : sm_lib/Frames and Transforms/Reference Frame
  Solid : sm_lib/Body Elements/Solid  InertiaType=Custom  Mass=smiData.Solid(1).mass  MassUnits=kg  CenterOfMass=smiData.Solid(1).CoM  CenterOfMassUnits=mm  MomentsOfInertia=smiData.Solid(1).MoI  MomentsOfInertiaUnits=kg*mm^2  ProductsOfInertia=smiData.Solid(1).PoI  ProductsOfInertiaUnits=kg*mm^2  BasedOnType=Density  Density=1000  DensityUnits=kg/m^3  DoExposeReferenceFrame=on  SerializedFrames=<Frames/>  GraphicType=FromGeometry  MarkerShape=Sphere  MarkerSize=10  GraphicVisPropType=SimpleVisualProperties  GraphicDiffuseColor=smiData.Solid(1).color  GraphicSpecularColor=[0.5 0.5 0.5 1.0]  GraphicAmbientColor=[0.15 0.15 0.15 1.0]  GraphicEmissiveColor=[0.0 0.0 0.0 1.0]  GraphicShininess=75  GraphicOpacity=smiData.Solid(1).opacity  GeometryShape=FromFile  RectangleSize=[1 1]  RectangleSizeUnits=m  BrickDimensions=[1 1 1]  BrickDimensionUnits=m  CylinderRadius=1  CylinderRadiusUnits=m  CylinderLength=1  CylinderLengthUnits=m  SphereRadius=1  SphereRadiusUnits=m  EllipsoidRadii=[1 1 1]  EllipsoidRadiiUnits=m  ExtrusionCrossSection=[1 1; -1 1; -1 -1; 1 -1]  ExtrusionCrossSectionUnits=m  ExtrusionLength=1  ExtrusionLengthUnits=m  PolygonNumSides=3  PolygonOuterRadius=1  PolygonOuterRadiusUnits=m  ExtGeomFileType=STEP  ExtGeomFileName=Link2_默认_sldprt.STEP  ExtGeomFileUnits=m  RevolutionCrossSection=[1 1; 1 -1; 2 -1; 2 1]  RevolutionCrossSectionUnits=m  RevolutionExtent=Full  RevolutionAngle=180  RevolutionAngleUnits=deg
  Transform : sm_lib/Frames and Transforms/Rigid Transform  TranslationMethod=Cartesian  TranslationStandardOffset=0  TranslationLengthUnit=mm  TranslationStandardAxis=+Z  TranslationCartesianOffset=smiData.RigidTransform(2).translation  TranslationROffset=0  TranslationROffsetUnits=m  TranslationZOffset=0  TranslationZOffsetUnits=m  TranslationThetaOffset=0  TranslationThetaOffsetUnits=deg  RotationMethod=ArbitraryAxis  RotationAngleUnits=rad  RotationStandardAxis=+Z  RotationAngle=smiData.RigidTransform(2).angle  RotationArbitraryAxis=smiData.RigidTransform(2).axis  FollAlignAxisA=+X  BaseAlignAxisA=+Y  FollAlignAxisB=+Y  BaseAlignAxisB=+Z  RotationSequenceAxes=FollowerAxes  RotationSequence=XYX  RotationSequenceAngles=[0 0 0]  RotationSequenceAnglesUnits=deg  RotationMatrix=[1 0 0; 0 1 0; 0 0 1]
  Transform1 : sm_lib/Frames and Transforms/Rigid Transform  TranslationMethod=Cartesian  TranslationStandardOffset=0  TranslationLengthUnit=mm  TranslationStandardAxis=+Z  TranslationCartesianOffset=smiData.RigidTransform(5).translation  TranslationROffset=0  TranslationROffsetUnits=m  TranslationZOffset=0  TranslationZOffsetUnits=m  TranslationThetaOffset=0  TranslationThetaOffsetUnits=deg  RotationMethod=ArbitraryAxis  RotationAngleUnits=rad  RotationStandardAxis=+Z  RotationAngle=smiData.RigidTransform(5).angle  RotationArbitraryAxis=smiData.RigidTransform(5).axis  FollAlignAxisA=+X  BaseAlignAxisA=+Y  FollAlignAxisB=+Y  BaseAlignAxisB=+Z  RotationSequenceAxes=FollowerAxes  RotationSequence=XYX  RotationSequenceAngles=[0 0 0]  RotationSequenceAnglesUnits=deg  RotationMatrix=[1 0 0; 0 1 0; 0 0 1]
  F : PMIOPort  Side=Left
  F1 : PMIOPort  Port=2  Side=Right
  connections:
  Solid/RConn1 -- ReferenceFrame/RConn1 -- Transform/LConn1 -- Transform1/LConn1
  Transform/RConn1 -- F/RConn1
  Transform1/RConn1 -- F1/RConn1

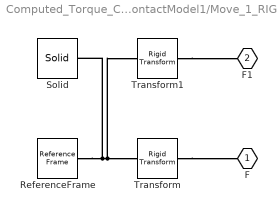
== system Computed_Torque_Control/SimscapeModelwithContactModel1/Move_1_RIGID ==
  ReferenceFrame : sm_lib/Frames and Transforms/Reference Frame
  Solid : sm_lib/Body Elements/Solid  InertiaType=Custom  Mass=smiData.Solid(5).mass  MassUnits=kg  CenterOfMass=smiData.Solid(5).CoM  CenterOfMassUnits=mm  MomentsOfInertia=smiData.Solid(5).MoI  MomentsOfInertiaUnits=kg*mm^2  ProductsOfInertia=smiData.Solid(5).PoI  ProductsOfInertiaUnits=kg*mm^2  BasedOnType=Density  Density=1000  DensityUnits=kg/m^3  DoExposeReferenceFrame=on  SerializedFrames=<Frames/>  GraphicType=FromGeometry  MarkerShape=Sphere  MarkerSize=10  GraphicVisPropType=SimpleVisualProperties  GraphicDiffuseColor=smiData.Solid(5).color  GraphicSpecularColor=[0.5 0.5 0.5 1.0]  GraphicAmbientColor=[0.15 0.15 0.15 1.0]  GraphicEmissiveColor=[0.0 0.0 0.0 1.0]  GraphicShininess=75  GraphicOpacity=smiData.Solid(5).opacity  GeometryShape=FromFile  RectangleSize=[1 1]  RectangleSizeUnits=m  BrickDimensions=[1 1 1]  BrickDimensionUnits=m  CylinderRadius=1  CylinderRadiusUnits=m  CylinderLength=1  CylinderLengthUnits=m  SphereRadius=1  SphereRadiusUnits=m  EllipsoidRadii=[1 1 1]  EllipsoidRadiiUnits=m  ExtrusionCrossSection=[1 1; -1 1; -1 -1; 1 -1]  ExtrusionCrossSectionUnits=m  ExtrusionLength=1  ExtrusionLengthUnits=m  PolygonNumSides=3  PolygonOuterRadius=1  PolygonOuterRadiusUnits=m  ExtGeomFileType=STEP  ExtGeomFileName=Move_默认_sldprt.STEP  ExtGeomFileUnits=m  RevolutionCrossSection=[1 1; 1 -1; 2 -1; 2 1]  RevolutionCrossSectionUnits=m  RevolutionExtent=Full  RevolutionAngle=180  RevolutionAngleUnits=deg
  Transform : sm_lib/Frames and Transforms/Rigid Transform  TranslationMethod=Cartesian  TranslationStandardOffset=0  TranslationLengthUnit=mm  TranslationStandardAxis=+Z  TranslationCartesianOffset=smiData.RigidTransform(6).translation  TranslationROffset=0  TranslationROffsetUnits=m  TranslationZOffset=0  TranslationZOffsetUnits=m  TranslationThetaOffset=0  TranslationThetaOffsetUnits=deg  RotationMethod=ArbitraryAxis  RotationAngleUnits=rad  RotationStandardAxis=+Z  RotationAngle=smiData.RigidTransform(6).angle  RotationArbitraryAxis=smiData.RigidTransform(6).axis  FollAlignAxisA=+X  BaseAlignAxisA=+Y  FollAlignAxisB=+Y  BaseAlignAxisB=+Z  RotationSequenceAxes=FollowerAxes  RotationSequence=XYX  RotationSequenceAngles=[0 0 0]  RotationSequenceAnglesUnits=deg  RotationMatrix=[1 0 0; 0 1 0; 0 0 1]
  Transform1 : sm_lib/Frames and Transforms/Rigid Transform  TranslationMethod=Cartesian  TranslationStandardOffset=0  TranslationLengthUnit=mm  TranslationStandardAxis=+Z  TranslationCartesianOffset=smiData.RigidTransform(7).translation  TranslationROffset=0  TranslationROffsetUnits=m  TranslationZOffset=0  TranslationZOffsetUnits=m  TranslationThetaOffset=0  TranslationThetaOffsetUnits=deg  RotationMethod=ArbitraryAxis  RotationAngleUnits=rad  RotationStandardAxis=+Z  RotationAngle=0  RotationArbitraryAxis=[0 0 1]  FollAlignAxisA=+X  BaseAlignAxisA=+Y  FollAlignAxisB=+Y  BaseAlignAxisB=+Z  RotationSequenceAxes=FollowerAxes  RotationSequence=XYX  RotationSequenceAngles=[0 0 0]  RotationSequenceAnglesUnits=deg  RotationMatrix=[1 0 0; 0 1 0; 0 0 1]
  F : PMIOPort  Side=Left
  F1 : PMIOPort  Port=2  Side=Right
  connections:
  Solid/RConn1 -- ReferenceFrame/RConn1 -- Transform/LConn1 -- Transform1/LConn1
  Transform/RConn1 -- F/RConn1
  Transform1/RConn1 -- F1/RConn1

== system Computed_Torque_Control/SimscapeModelwithContactModel1/Origin ==
  ReferenceFrame : sm_lib/Frames and Transforms/Reference Frame
  F : PMIOPort  Side=Left
  connections:
  ReferenceFrame/RConn1 -- F/RConn1

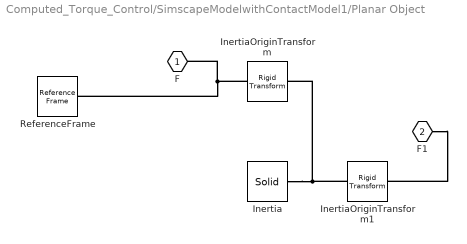
== system Computed_Torque_Control/SimscapeModelwithContactModel1/Planar Object ==
  Inertia : sm_lib/Body Elements/Solid  InertiaType=Custom  Mass=1e8  MassUnits=kg  CenterOfMass=[0, 0, 0]  CenterOfMassUnits=m  MomentsOfInertia=[1e-08, 1e-08, 1e-08]  MomentsOfInertiaUnits=kg*m^2  ProductsOfInertia=[1e-08, 1e-08, 1e-08]  ProductsOfInertiaUnits=kg*m^2  BasedOnType=Density  Density=1000  DensityUnits=kg/m^3  DoExposeReferenceFrame=on  SerializedFrames=<Frames/>  GraphicType=FromGeometry  MarkerShape=Sphere  MarkerSize=10  GraphicVisPropType=SimpleVisualProperties  GraphicDiffuseColor=[0.5 0.5 0.5]  GraphicSpecularColor=[0.5 0.5 0.5 1.0]  GraphicAmbientColor=[0.15 0.15 0.15 1.0]  GraphicEmissiveColor=[0.0 0.0 0.0 1.0]  GraphicShininess=75  GraphicOpacity=1  GeometryShape=Brick  RectangleSize=[1 1]  RectangleSizeUnits=m  BrickDimensions=[0.1 1 1]  BrickDimensionUnits=m  CylinderRadius=1  CylinderRadiusUnits=m  CylinderLength=1  CylinderLengthUnits=m  SphereRadius=1  SphereRadiusUnits=m  EllipsoidRadii=[1 1 1]  EllipsoidRadiiUnits=m  ExtrusionCrossSection=[1 1; -1 1; -1 -1; 1 -1]  ExtrusionCrossSectionUnits=m  ExtrusionLength=1  ExtrusionLengthUnits=m  PolygonNumSides=3  PolygonOuterRadius=1  PolygonOuterRadiusUnits=m  ExtGeomFileType=STEP  ExtGeomFileUnits=m  RevolutionCrossSection=[1 1; 1 -1; 2 -1; 2 1]  RevolutionCrossSectionUnits=m  RevolutionExtent=Full  RevolutionAngle=180  RevolutionAngleUnits=deg
  InertiaOriginTransform : sm_lib/Frames and Transforms/Rigid Transform  TranslationMethod=Cartesian  TranslationStandardOffset=0  TranslationLengthUnit=m  TranslationStandardAxis=+Z  TranslationCartesianOffset=[0.3, 0, -0.05]  TranslationROffset=0  TranslationROffsetUnits=m  TranslationZOffset=0  TranslationZOffsetUnits=m  TranslationThetaOffset=0  TranslationThetaOffsetUnits=deg  RotationMethod=StandardAxis  RotationAngleUnits=deg  RotationStandardAxis=+Y  RotationAngle=90  RotationArbitraryAxis=[0 0 1]  FollAlignAxisA=+X  BaseAlignAxisA=+Y  FollAlignAxisB=+Y  BaseAlignAxisB=+Z  RotationSequenceAxes=BaseAxes  RotationSequence=XYZ  RotationSequenceAngles=[0, -1, 0]  RotationSequenceAnglesUnits=rad  RotationMatrix=[1 0 0; 0 -1 0; 0 0 -1]
  InertiaOriginTransform1 : sm_lib/Frames and Transforms/Rigid Transform  TranslationMethod=None  TranslationStandardOffset=0  TranslationLengthUnit=m  TranslationStandardAxis=+Z  TranslationCartesianOffset=[0.3, 0, -0.05]  TranslationROffset=0  TranslationROffsetUnits=m  TranslationZOffset=0  TranslationZOffsetUnits=m  TranslationThetaOffset=0  TranslationThetaOffsetUnits=deg  RotationMethod=RotationMatrix  RotationAngleUnits=deg  RotationStandardAxis=+Y  RotationAngle=90  RotationArbitraryAxis=[0 0 1]  FollAlignAxisA=+X  BaseAlignAxisA=+Y  FollAlignAxisB=+Y  BaseAlignAxisB=+Z  RotationSequenceAxes=BaseAxes  RotationSequence=XYZ  RotationSequenceAngles=[0, -1, 0]  RotationSequenceAnglesUnits=rad  RotationMatrix=[0 0 -1;0 -1 0;-1 0 0]
  ReferenceFrame : sm_lib/Frames and Transforms/Reference Frame
  F : PMIOPort  Side=Left
  F1 : PMIOPort  Port=2  Side=Left
  connections:
  Inertia/RConn1 -- InertiaOriginTransform1/LConn1 -- InertiaOriginTransform/RConn1
  ReferenceFrame/RConn1 -- InertiaOriginTransform/LConn1 -- F/RConn1
  F1/RConn1 -- InertiaOriginTransform1/RConn1

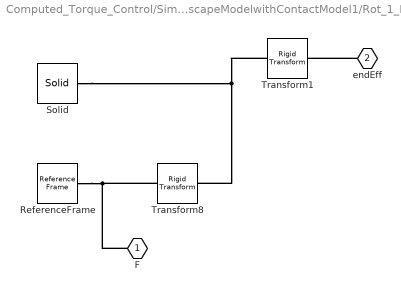
== system Computed_Torque_Control/SimscapeModelwithContactModel1/Rot_1_RIGID ==
  ReferenceFrame : sm_lib/Frames and Transforms/Reference Frame
  Solid : sm_lib/Body Elements/Solid  InertiaType=Custom  Mass=smiData.Solid(2).mass  MassUnits=kg  CenterOfMass=smiData.Solid(2).CoM  CenterOfMassUnits=mm  MomentsOfInertia=smiData.Solid(2).MoI  MomentsOfInertiaUnits=kg*mm^2  ProductsOfInertia=smiData.Solid(2).PoI  ProductsOfInertiaUnits=kg*mm^2  BasedOnType=Density  Density=1000  DensityUnits=kg/m^3  DoExposeReferenceFrame=on  SerializedFrames=<Frames/>  GraphicType=FromGeometry  MarkerShape=Sphere  MarkerSize=10  GraphicVisPropType=SimpleVisualProperties  GraphicDiffuseColor=smiData.Solid(2).color  GraphicSpecularColor=[0.5 0.5 0.5 1.0]  GraphicAmbientColor=[0.15 0.15 0.15 1.0]  GraphicEmissiveColor=[0.0 0.0 0.0 1.0]  GraphicShininess=75  GraphicOpacity=smiData.Solid(2).opacity  GeometryShape=FromFile  RectangleSize=[1 1]  RectangleSizeUnits=m  BrickDimensions=[1 1 1]  BrickDimensionUnits=m  CylinderRadius=1  CylinderRadiusUnits=m  CylinderLength=1  CylinderLengthUnits=m  SphereRadius=1  SphereRadiusUnits=m  EllipsoidRadii=[1 1 1]  EllipsoidRadiiUnits=m  ExtrusionCrossSection=[1 1; -1 1; -1 -1; 1 -1]  ExtrusionCrossSectionUnits=m  ExtrusionLength=1  ExtrusionLengthUnits=m  PolygonNumSides=3  PolygonOuterRadius=1  PolygonOuterRadiusUnits=m  ExtGeomFileType=STEP  ExtGeomFileName=Rot_默认_sldprt.STEP  ExtGeomFileUnits=m  RevolutionCrossSection=[1 1; 1 -1; 2 -1; 2 1]  RevolutionCrossSectionUnits=m  RevolutionExtent=Full  RevolutionAngle=180  RevolutionAngleUnits=deg
  Transform1 : sm_lib/Frames and Transforms/Rigid Transform  TranslationMethod=StandardAxis  TranslationStandardOffset=0  TranslationLengthUnit=mm  TranslationStandardAxis=+Z  TranslationCartesianOffset=smiData.RigidTransform(8).translation  TranslationROffset=0  TranslationROffsetUnits=m  TranslationZOffset=0  TranslationZOffsetUnits=m  TranslationThetaOffset=0  TranslationThetaOffsetUnits=deg  RotationMethod=RotationSequence  RotationAngleUnits=rad  RotationStandardAxis=+Z  RotationAngle=smiData.RigidTransform(8).angle  RotationArbitraryAxis=smiData.RigidTransform(8).axis  FollAlignAxisA=+X  BaseAlignAxisA=+Y  FollAlignAxisB=+Y  BaseAlignAxisB=+Z  RotationSequenceAxes=FollowerAxes  RotationSequence=XYX  RotationSequenceAngles=[0 0 0]  RotationSequenceAnglesUnits=deg  RotationMatrix=[1 0 0; 0 -1 0; 0 0 -1]
  Transform8 : sm_lib/Frames and Transforms/Rigid Transform  TranslationMethod=Cartesian  TranslationStandardOffset=0  TranslationLengthUnit=mm  TranslationStandardAxis=+Z  TranslationCartesianOffset=[0 0 -330]  TranslationROffset=0  TranslationROffsetUnits=m  TranslationZOffset=0  TranslationZOffsetUnits=m  TranslationThetaOffset=0  TranslationThetaOffsetUnits=deg  RotationMethod=RotationSequence  RotationAngleUnits=rad  RotationStandardAxis=+Z  RotationAngle=90  RotationArbitraryAxis=[0 1 0]  FollAlignAxisA=+X  BaseAlignAxisA=+Y  FollAlignAxisB=+Y  BaseAlignAxisB=+Z  RotationSequenceAxes=FollowerAxes  RotationSequence=XYX  RotationSequenceAngles=[0 0 0]  RotationSequenceAnglesUnits=deg  RotationMatrix=[1 0 0; 0 1 0; 0 0 1]
  F : PMIOPort  Side=Left
  endEff : PMIOPort  Port=2  Side=Right
  connections:
  endEff/RConn1 -- Transform1/RConn1
  ReferenceFrame/RConn1 -- Transform8/LConn1 -- F/RConn1
  Transform1/LConn1 -- Solid/RConn1 -- Transform8/RConn1

== system Computed_Torque_Control/SimscapeModelwithContactModel1/Signal Builder ==
  Demux : Demux  Tag=STV Demux  Outputs=1
  FromWs : FromWorkspace  Tag=STV FromWs  VariableName=tuvar  SampleTime=0
      SigBuilderData=|
      | common.afterFinalStr = 'Extrapolate'
      | common.sampleTime = 0
      | dataSet.timeRange = [0 10]
      | dataSet.name = 'Group 1'
      | sbobj.Groups.Name = 'Group 1'
      | sbobj.Groups.Signals.Name = 'Signal 1'
      | sbobj.Groups.Signals.XData = [0 2 4 6 10]
      | sbobj.Groups.Signals.YData = [0 0 39.8 0 0]
  Signal 1 : Outport  Tag=STV Outport
  wires:
  Demux/1 -> Signal 1/1
  FromWs/1 -> Demux/1

== system Computed_Torque_Control/SimscapeModelwithContactModel1/Signal Builder1 ==
  Demux : Demux  Tag=STV Demux  Outputs=1
  FromWs : FromWorkspace  Tag=STV FromWs  VariableName=tuvar  SampleTime=0
      SigBuilderData=|
      | common.afterFinalStr = 'Extrapolate'
      | common.sampleTime = 0
      | dataSet.timeRange = [0 10]
      | dataSet.name = 'Group 1'
      | sbobj.Groups.Name = 'Group 1'
      | sbobj.Groups.Signals.Name = 'Signal 1'
      | sbobj.Groups.Signals.XData = [0 2 4 10]
      | sbobj.Groups.Signals.YData = [0 30 0 0]
  Signal 1 : Outport  Tag=STV Outport
  wires:
  Demux/1 -> Signal 1/1
  FromWs/1 -> Demux/1
